simulink model "contrPIDbas"  (R2021b)
settings: Solver=VariableStepAuto  StartTime=0.0  StopTime=11  RelTol=1e-3
settings Model: Creator=axel_  LastModifiedBy=axel_

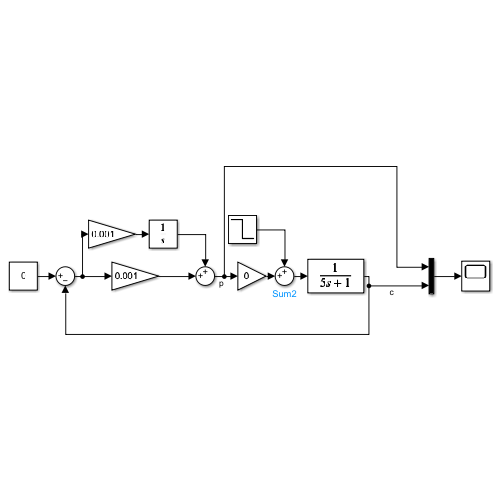
[thumbnail: Simulink's stored preview of the top-level diagram]
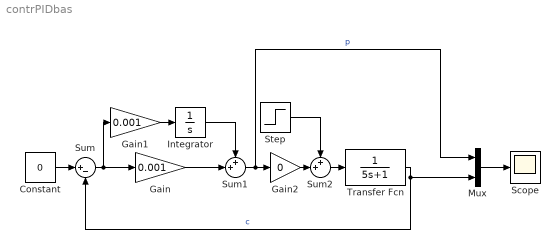
== system contrPIDbas ==
  Constant : Constant  Value=0
  Gain : Gain  Gain=0.001
  Gain1 : Gain  Gain=0.001
  Gain2 : Gain  Gain=0
  Integrator : Integrator
  Mux : Mux  Inputs=2
  Scope : Scope
  Step : Step  After=-1500  SampleTime=0
  Sum : Sum  Inputs=|+-
  Sum1 : Sum  Inputs=++|
  Sum2 : Sum  Inputs=++|
  Transfer Fcn : TransferFcn  Denominator=[5 1]
  wires:
  Transfer Fcn/1 -> Mux/2, Sum/2  "c"
  Gain1/1 -> Integrator/1
  Sum/1 -> Gain/1, Gain1/1
  Integrator/1 -> Sum1/1
  Gain/1 -> Sum1/2
  Sum1/1 -> Mux/1, Gain2/1  "p"
  Gain2/1 -> Sum2/2
  Sum2/1 -> Transfer Fcn/1
  Step/1 -> Sum2/1
  Constant/1 -> Sum/1
  Mux/1 -> Scope/1
